simulink model "Sim6_lim_current_LCL"  (R2018b)
settings: Solver=ode1  StartTime=0.0  StopTime=5  FixedStep=Time_Step  MaxStep=1e-4  RelTol=1e-3
undefined symbols (not defined in the file): Bxx_GenericVoltageSource, C_line, Lg, Rg, Source_Lib, Theta0, Time_Step, Un, V0, VSC01_id0
libraries: powerlib x34, Control_Lib x7, powerlib_meascontrol x4, simulink x4
(part 1 of 2)
settings Model: Creator=Frederic_Colas  LastModifiedBy=fcolas
settings OptimizationCC: LifeSpan=inf
settings DebuggingCC: UnconnectedInputMsg=none  UnconnectedOutputMsg=none  UnconnectedLineMsg=none  SFExecutionAtInitializationDiag=none
settings HardwareCC: ProdBitPerSizeT=32  ProdBitPerPtrDiffT=32  ProdWordSize=32  ProdHWDeviceType=Specified
settings SFSimCC: SimUseLocalCustomCode=off
settings RTWCC: RTWUseLocalCustomCode=off
settings CodeAppCC: StateflowObjectComments=on
settings SimscapeCC: SimscapeNormalizeSystem=off

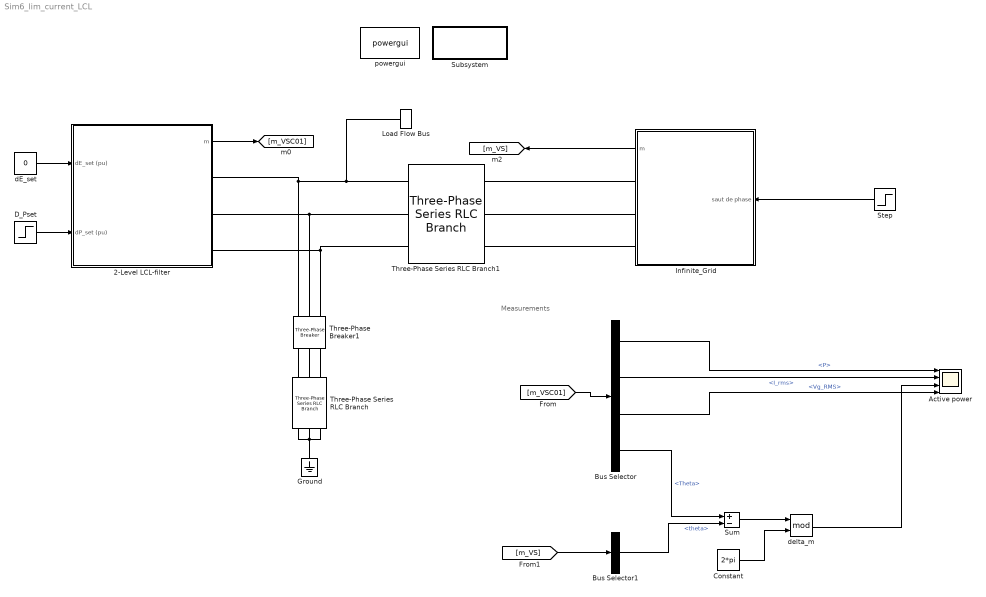
== system Sim6_lim_current_LCL ==
  note: Measurements
  2-Level LCL-filter : Subsystem  AncestorBlock=GFo_Lib/2-Level LCL-filter  mask(VSC){fn=50, Sn=1000e6, Pn=1000e6, Udcn=640e3, Time_Step=Time_Step, bridge_type=Average (no switches), fpwm=4e3, Un1=320e3, Un2=400e3, Rt_pu=0.005, Lt_pu=0.15, Rm_pu=500, Lm_pu=500, Lf_pu=0.15, Rf_pu=0.005, Cf_pu=0.066, H_DC=40, Tr_PLL=10, Val_Freq_Support=on, Val_gamma=on, R_percent=4, Rv=0.009, W_TVR=60, I_max_VI_pu=1.1, DX_DR=5, Kp_Rvi_pu=0.676, RLCL_D=0.7, f_damping=100, I_max_pu=1.15, Tr_I_max=10, Advanced=on, gainpopup=With Inertia, f_Inertia_Less=3, zeta_Inertia_Less=1, Param_Inertia=PI, H_GFo=5, zeta_GFo=0.7, LFpopup=PQ, P0=0.5, Q0=-1.3878e-17, V0=1.0022, Theta0=1.429}
      mask prompts: fn "Nominal Frequency (Hz)"; Sn "Nominal Apparent Power (VA)"; Pn "Nominal Power (W)"; Udcn "Nominal DC Voltage (V)"; Time_Step "Sample Time (s)"; bridge_type "Bridge Type"; fpwm "PWM frequency (Hz)"; Un1 "VSC side Nominal Ph-Ph Voltage (V)"; Un2 "Grid side Nominal Ph-Ph Voltage (V)"; Rt_pu "R (pu)"; Lt_pu "L (pu)"; Rm_pu "Rm (pu)"; Lm_pu "Lm (pu)"; Lf_pu "Lf (pu)"; Rf_pu "Rf (pu)"; Cf_pu "Cf (pu)"; H_DC "DC inertia (ms)"; Tr_PLL "Time response (ms)"; Val_Freq_Support "Frequency Support"; Val_gamma "gamma activation"; R_percent "Droop Gain (%)"; Rv "Damping Resistance (Rv)"; W_TVR "Dr filter"; I_max_VI_pu "Current Threshold (pu)"; Kp_Rvi_pu "Kp_Rvi"; RLCL_D "LC Damping Resistance (pu)"; f_damping "Cut-off Frequency (Hz)"; I_max_pu "I max (pu)"; Tr_I_max "Current Loop time response (ms)"; gainpopup "Strategy"; f_Inertia_Less "Bandwidth (Hz)"; zeta_Inertia_Less "Damping"; H_GFo "Inertia H (s)"; zeta_GFo "Damping Ratio"; P0 "Initial Active Power (pu)"; Q0 "Initial Reactive Power (pu)"; V0 "Initial Voltage (pu)"; Theta0 "Initial Angle (°)"
      mask init:
      | % Base values
      |     % 1 = VSC side
      |     % 2 = grid side
      |     fb = fn;
      |     Pb = Pn;
      |     cos_phi_n = Pn/Sn;
      |     Sb = Pb/cos_phi_n;
      |     Vn1 = Un1/sqrt(3);
      |     Vb1 = Vn1;
      |     Vn2 = Un2/sqrt(3);
      |     Vb2 = Vn2;
      |     Ib1 = Sb / (3*Vb1);
      |     Ib2 = Sb / (3*Vb2);
      |     Zb = (3*Vb1^2)/Sb;
      |     wb = 2*pi*fb;  wb_pu=1;
      |     Lb = Zb/wb;
      |     Cb = 1/(Zb*wb);
      |     
      | % Grid-Forming control tuning
      |     % Inertia Less
      |     wn_Inertia_Less = 2*pi*f_Inertia_Less;
      |     Ki_Inertia_Less = Lt_pu*wn_Inertia_Less^2/wb;
      |     Kp_Inertia_Less = 2*zeta_Inertia_Less*wn_Inertia_Less*Lt_pu/wb;
      |     
      |     % With Inertia
      |     Kc = 1/Lf_pu;
      |     Kg = 1/Lt_pu;
      |     %H_Gfo = 3;
      |     %wn = sqrt(wb*Kc*Kg/(2*H_Gfo*(Kc+Kg)));
      |     kp_GFo = zeta_GFo*sqrt(2*(Kc+Kg)/(H_GFo*wb*Kc*Kg));
      |     kd = 2*H_GFo*kp_GFo*Kc*wb;
      |   
      | % PLL derivation of the parameters
      |     wn_PLL=5/Tr_PLL;
      |     zeta_PLL = 1;
      |     Kp_PLL_pu = 2*zeta_PLL*wn_PLL/wb;
      |     Ki_PLL_pu = wn_PLL^2/wb;
      |     
      |     
      |     % VI calculation
      | 
      | 
      |   A_VI = (1 + 1/DX_DR^2);
      |   B_VI = 2*Lt_pu;
      |   C_VI = Lt_pu^2 - 1/I_max_VI_pu^2;
      |   
      |   Delta_VI = B_VI^2 - 4*A_VI*C_VI;
      |   
      |   X1_VI = (-B_VI + sqrt(Delta_VI))/(2*A_VI);
      |   Kp_Rvi_pu = X1_VI/(DX_DR*(-1+I_max_VI_pu));
      |   
      |   
      | % Set the chosen strategy
      |     if (gainpopup == 1)
      |         Chosen_Strategy = 1;
      |     elseif (gainpopup == 2)
      |         if (Param_Inertia == 1)
      |             Chosen_Strategy = 2;
      |         elseif (Param_Inertia == 2)
      |             Chosen_Strategy = 3;
      |         end
      |     end
      |     %Chosen_Strategy = 2;
      |     
      | % Set the frequency droop gain
      |     R = R_percent/100;
      | 
      | % Compute the delay compensation between control and power parts
      |     if (Time_Step == -1)
      |         Solver_Time_Step = 0;
      |     else
      |         Solver_Time_Step = Time_Step;
      |     end
      | 
      | % Compute Initial Voltage of VSC 
      | %   from steady-state output transformer model and Loadflow result
      |     
      |     %Initialize correctly the LoadFlow bus parameters connected to PCC
      |     VLF = V0;
      |     ThetaLF = Theta0;
      |     if (LFpopup == 'PQ')
      |         VLF = 1;
      |         ThetaLF = 0;
      |     elseif (LFpopup == 'PV')
      |         VLF = V0;
      |         ThetaLF = 0;        
      |     end
      |     %set_param([gcb '/Load Flow Bus'],'Vref',num2str(VLF),'Vangle',num2str(ThetaLF));
      | 
      |     % steady-state model of output transformer
      |     R1_pu = Rt_pu/2;
      |     L1_pu = Lt_pu/2;
      |     R2_pu = Rt_pu/2;
      |     L2_pu = Lt_pu/2;
      |     X1_pu = L1_pu;
      |     X2_pu = L2_pu;
      |     Xm_pu = Lm_pu;
      |     wb_pu = 1;
      |     
      |     Zm_pu = 1/(1/Rm_pu+1/(1i*Xm_pu));
      |     S0=P0+1i*Q0;
      |     I2 = conj(S0)/(V0);
      |     Vm = (R2_pu+1i*X2_pu)*I2 + V0;
      |     Im = Vm/Zm_pu;
      |     I1 = I2 + Im;
      |     V1 = (R1_pu+1i*X1_pu) * I1 + Vm;
      |     
      |     Eg0 = abs(V1); % compute initial Eg value
      |     Theta_m0 = angle(V1) * 180/pi+Theta0;
      |     
      |     %Steady-state model of LC Filter
      |     Is = I1 + 1i*Cf_pu*V1;
      |     Theta_Is = angle(Is) * 180/pi+Theta0;
      |     Vm = (1i*Lf_pu+Rf_pu)*Is+ V1;  %  
      |     
      | % Generate string to display LF results on Mask
      |     %str_tmp = fprintf("Vvsc0 = %d, Theta_vsc0 = %d°",Vvsc0,Theta_vsc0);
      |     mo = get_param(gcb,'MaskObject');
      |     mo.getDialogControl('LF_pcc_str').Prompt = ['V0 = ', num2str(V0),' pu, Angle = ', num2str(Theta0),'°'];
      |     mo.getDialogControl('LF_pcc_Power_str').Prompt = ['P0 = ', num2str(P0),' pu, Q0 = ', num2str(Q0),' pu'];
      |     %set_param([gcb],'LF_str',str_tmp);
      |  %GRD00_Theta0 = Theta0;
      |  % Initial current and voltage states calculation 
      |  
      | % Given Setpoint in PV bus
      |  
      | Vg0_d=V0*cos(Theta0*pi/180-Theta_m0*pi/180);
      | Vg0_q=V0*sin(Theta0*pi/180-Theta_m0*pi/180);
      | Vg0_dq = [Vg0_d ;Vg0_q; 0];
      |  
      | % Initial state of AC grid current : Ig0dq
      | 
      | Theta_I2 = angle(I2) * 180/pi + Theta0;
      | Ig0_d = abs(I2)*cos(Theta_I2*pi/180-Theta_m0*pi/180);
      | Ig0_q = abs(I2)*sin(Theta_I2*pi/180-Theta_m0*pi/180);
      | Ig0_dq = [Ig0_d; Ig0_q; 0];
      |  
      | % Initial state of capacitor voltage : eg0dq
      | 
      | Eg0_d = Eg0;
      | Eg0_q = 0;
      | Eg0_dq = [Eg0; 0; 0];
      |  
      | % Initial state of VSC Current : Is0dq
      | 
      | Is0_d = abs(Is) * cos(Theta_Is*pi/180-Theta_m0*pi/180);
      | Is0_q = abs(Is) * sin(Theta_Is*pi/180-Theta_m0*pi/180);
      | Is0_dq = [Is0_d; Is0_q; 0];
      | 
      | % Initial state of Modulation Voltage : Vm0dq
      | 
      | Vvsc0 = abs(Vm);
      | Theta_vsc0 = angle(Vm)*180/pi + Theta0;
      | Vm0_d = Vvsc0 * cos(Theta_vsc0*pi/180-Theta_m0*pi/180);
      | Vm0_q = Vvsc0 * sin(Theta_vsc0*pi/180-Theta_m0*pi/180);
      |  
      | Va0 = sqrt(2)*Vb1*Vvsc0*sin(Theta_vsc0*pi/180);
      | Vb0 = sqrt(2)*Vb1*Vvsc0*sin(Theta_vsc0*pi/180-2*pi/3);
      | Vc0 = sqrt(2)*Vb1*Vvsc0*sin(Theta_vsc0*pi/180+2*pi/3);
      | Vabc0 = [Va0 Vb0 Vc0];
      |  
      | mo.getDialogControl('LF_vsc_str').Prompt = ['V0 = ', num2str(Eg0),' pu, Angle = ', num2str(Theta_m0),'°'];
      settings: OpenFcn=|
      | NameStr = get_param(gcb,'Name');
      | open_system(gcbh, 'Mask');
      | 
      | h2AllOpenDlgs = DAStudio.ToolRoot.getOpenDialogs;
      | 
      | for i=1:length(h2AllOpenDlgs)
      |     try
      |          %disp(h2AllOpenDlgs(i).getSource.getBlock.Name);
      |         Dialog_block_name = h2AllOpenDlgs(i).getSource.getBlock.Name;
      |          %strcmp(Dialog_block_name, NameStr),
      |         if (strcmp(h2AllOpenDlgs(i).getSource.getBlock.Name, NameStr))
      |             iPos = h2AllOpenDlgs(i).position;
      |             h2AllOpenDlgs(i).position = [iPos(1)   iPos(2)   iPos(3)*1.6   iPos(4)];
      |         end
      |     end
      | end
      mask TypeOptions bridge_type: Average (no switches) | Detailed (switches included)
      mask Callback bridge_type:
      | % Get the mask parameter values. This is a cell
      | %   array of character vectors.
      | maskStr = get_param(gcb,'bridge_type');
      | p=Simulink.Mask.get(gcb);
      | 
      | % The pop-up menu is the first mask parameter.
      | %   Check the value selected in the pop-up
      | if strcmp(maskStr,'Average (no switches)'),
      | 
      |     % Set the visibility of both parameters on when
      |     %   User-defined is selected in the pop-up.
      |     p.getDialogControl('pwm_box').Visible='off';
      |     set_param([gcb '/Bridge_Model/Average'],'Commented','off');
      |     set_param([gcb '/Bridge_Model/Detailed'],'Commented','on');
      | 
      | 
      | elseif strcmp(maskStr,'Detailed (switches included)'),
      | 
      |     % Set the visibility of both parameters on when
      |     %   User-defined is selected in the pop-up.
      |     p.getDialogControl('pwm_box').Visible='on';
      |     set_param([gcb '/Bridge_Model/Average'],'Commented','on');
      |     set_param([gcb '/Bridge_Model/Detailed'],'Commented','off');
      | 
      | end
      mask Callback Advanced:
      | % Get the mask parameter values. This is a cell
      | %   array of character vectors.
      | maskStr = get_param(gcb,'Advanced');
      | p=Simulink.Mask.get(gcb);
      | 
      | % The pop-up menu is the first mask parameter.
      | %   Check the value selected in the pop-up
      | if strcmp(maskStr,'on'),
      | 
      |     % Set the visibility of both parameters on when
      |     %   User-defined is selected in the pop-up.
      |     p.getDialogControl('TVR').Visible='on';
      |     p.getDialogControl('TVI').Visible='on';
      |     p.getDialogControl('LC_Filter').Visible='on';
      |     p.getDialogControl('Current_Sat').Visible='on';
      |     %p.getDialogControl('Param_Strat_3').Visible='off';
      | 
      | 
      | else
      | 
      |     % Set the visibility of both parameters on when
      |     %   User-defined is selected in the pop-up.
      |     p.getDialogControl('TVR').Visible='off';
      |     p.getDialogControl('TVI').Visible='off';
      |     p.getDialogControl('LC_Filter').Visible='off';
      |     p.getDialogControl('Current_Sat').Visible='off';
      |     %p.getDialogControl('Param_Strat_3').Visible='off';
      | 
      | end
      mask TypeOptions gainpopup: Inertia Less | With Inertia
      mask Callback gainpopup:
      | % Get the mask parameter values. This is a cell
      | %   array of character vectors.
      | maskStr = get_param(gcb,'gainpopup');
      | p=Simulink.Mask.get(gcb);
      | 
      | % The pop-up menu is the first mask parameter.
      | %   Check the value selected in the pop-up
      | if strcmp(maskStr,'Inertia Less'),
      | 
      |     % Set the visibility of both parameters on when
      |     %   User-defined is selected in the pop-up.
      |     p.getDialogControl('No_Inertia').Visible='on';
      |     p.getDialogControl('Inertia').Visible='off';
      |     %p.getDialogControl('Param_Strat_3').Visible='off';
      | 
      | 
      | elseif strcmp(maskStr,'With Inertia'),
      | 
      |     % Set the visibility of both parameters on when
      |     %   User-defined is selected in the pop-up.
      |     p.getDialogControl('No_Inertia').Visible='off';
      |     p.getDialogControl('Inertia').Visible='on';
      |     %p.getDialogControl('Param_Strat_3').Visible='off';
      | 
      | 
      |     % Turn off the visibility of the Value field
      |     %   when User-defined is not selected.
      | 
      | else
      | 
      |     % Set the visibility of both parameters on when
      |     %   User-defined is selected in the pop-up.
      |     p.getDialogControl('No_Inertia').Visible='off';
      |     p.getDialogControl('Inertia').Visible='off';
      |     %p.getDialogControl('Param_Strat_3').Visible='off';
      | 
      | end
      mask TypeOptions Param_Inertia: VSM | PI
      mask TypeOptions LFpopup: Swing | PQ | PV
      mask Callback LFpopup:
      | % Get the mask parameter values. This is a cell
      | %   array of character vectors.
      | maskStr = get_param(gcb,'LFpopup');
      | p=Simulink.Mask.get(gcb);
      | 
      | % The pop-up menu is the first mask parameter.
      | %   Check the value selected in the pop-up
      | if strcmp(maskStr,'Swing'),
      | 
      |     % Set the visibility of both parameters on when
      |     %   User-defined is selected in the pop-up.
      |     p.getParameter('P0').Visible='off';
      |     p.getParameter('Q0').Visible='off';
      |     p.getParameter('V0').Visible='on';
      |     p.getParameter('Theta0').Visible='on';
      |     set_param([gcb '/Source_For_LF'],'BusType','swing');
      | 
      | elseif strcmp(maskStr,'PQ'),
      | 
      |     % Set the visibility of both parameters on when
      |     %   User-defined is selected in the pop-up.
      |     p.getParameter('P0').Visible='on';
      |     p.getParameter('Q0').Visible='on';
      |     %p.getParameter('V0').Value='1';
      |     %set_param(gcb,'V0','1');
      |     p.getParameter('V0').Visible='off';
      |     p.getParameter('Theta0').Visible='off';
      |     set_param([gcb '/Source_For_LF'],'BusType','PQ');
      | 
      |     % Turn off the visibility of the Value field
      |     %   when User-defined is not selected.
      | else
      | 
      |     % Set the visibility of both parameters on when
      |     %   User-defined is selected in the pop-up.
      |     p.getParameter('P0').Visible='on';
      |     p.getParameter('Q0').Visible='off';
      |     p.getParameter('V0').Visible='on';
      |     p.getParameter('Theta0').Visible='off';
      |     set_param([gcb '/Source_For_LF'],'BusType','PV');
      | 
      | end
      mask DialogControl Nominal_Param Prompt: Nominal Value
      mask DialogControl Container20 Prompt: Passive Components
      mask DialogControl Container31 Prompt: Transformer
      mask DialogControl Container32 Prompt: Filter
      mask DialogControl Container35 Prompt: DC Link
      mask DialogControl Control_Param Prompt: Control Parameter
      mask DialogControl Container13 Prompt: PLL
      mask DialogControl Container14 Prompt: Frequency Support
      mask DialogControl TVR Prompt: Transient Virtual Resistor
      mask DialogControl TVI Prompt: Virtual Impedance
      mask DialogControl LC_Filter Prompt: LC Filter
      mask DialogControl Current_Sat Prompt: Current Limitation
      mask DialogControl Container18 Prompt: Control Strategy
      mask DialogControl LF_Param Prompt: Loadflow
      mask DialogControl Control4 Prompt: Initial Operating Point
      mask DialogControl Container24 Prompt: VSC side
      mask DialogControl LF_vsc_str Prompt: V0 = 1.0076 pu, Angle = 5.6968°
      mask DialogControl Container25 Prompt: PCC
      mask DialogControl LF_pcc_str Prompt: V0 = 1.0022 pu, Angle = 1.429°
      mask DialogControl LF_pcc_Power_str Prompt: P0 = 0.5 pu, Q0 = -1.3878e-17 pu
      mask DialogControl UpdateLoadflow Prompt: Update Loadflow
      mask DialogControl UpdateLoadflow Callback: LoadFlow_VSC
      mask Display:
      | disp('LCL-Filter');
      | port_label('input',1,'dE_set (pu)');
      | port_label('input',2,'dP_set (pu)');
      | port_label('output',1,'m');
      | port_label('rconn',1,'A');
      | port_label('rconn',2,'B');
      | port_label('rconn',3,'C');
  Active power : Scope  NumInputPorts=4
  Bus Selector : BusSelector  OutputSignals=P,VI.I_rms,V.Vg_RMS,Theta
  Bus Selector1 : BusSelector  OutputSignals=Theta.theta
  Constant : Constant  Value=2*pi
  D_Pset : Step  After=0  SampleTime=0
  Ground : powerlib/Elements/Ground  LConnTagsString=a
  Infinite_Grid : Subsystem  AncestorBlock=Source_Lib/Bxx_GenericVoltageSource  mask(GenericVoltageSource){SourceNature_str=INFINITE, fn=50, Sn=1e9, Un=Un, LFpopup=Swing, P0=-498595539.7375, Q0=12437610.3184, V0_pu=1, U0=20000, Theta0_deg=0, H_s=5, DroopOnOff=on, R_percent=4, TN=1, TD=2}
      mask prompts: SourceNature_str "Nature of the voltage source"; fn "Nominal frequency fn [Hz]"; Sn "Nominal apparent power Sn [VA]"; Un "Nominal voltage Un [V RMS Ph2Ph]"; P0 "Active power P0 [W]"; Q0 "Reactive power Q0 [VAR]"; V0_pu "Initial pu voltage V0_pu [pu]"; U0 "Initial voltage U0 [Vrms Ph2Ph]"; Theta0_deg "Initial angle (°)"; H_s "Inertia H [s]"; DroopOnOff "Frequency DROOP activation"; R_percent "Droop gain Kp [%]"; TN "Network time constant Lead [s]"; TD "Network time constant Lag [s]"
      mask init:
      | % Update Name of LF bus for internal purpose
      | NameStr = [get_param(gcb,'Name')];% '_LF'];
      | set_param([gcb '/Load Flow Bus'],'ID',NameStr);  
      | 
      | % Base specification
      | fb = fn;                % [Hz] base frequency
      | Sb = Sn;                % [VA] base power
      | Ub = Un;                % [V] base ph2ph voltage
      | Vb = Un/sqrt(3);        % [V] base ph2N voltage
      | Ib = Sb/(3*Vb);         % [A] base current
      | Zb = Vb*Ib;             % [Ohm] base impedance
      | 
      | % Set the frequency droop gain
      | R = R_percent / 100;
      | 
      | %Initialize correctly the LoadFlow bus parameters connected to PCC
      |     VLF = V0_pu;
      |     ThetaLF = Theta0_deg;
      |     if (LFpopup == 'PQ')
      |         VLF = 1;
      |         ThetaLF = 0;
      |     elseif (LFpopup == 'PV')
      |         VLF = V0_pu;
      |         ThetaLF = 0;        
      |     end
      |     set_param([gcb '/Load Flow Bus'],'Vref',num2str(VLF),'Vangle',num2str(ThetaLF));
      | 
      | 
      | % Update mask display:
      | % mo = get_param(gcb,'MaskObject');
      mask TypeOptions SourceNature_str: INFINITE | INERTIAL
      mask Callback SourceNature_str:
      | % Get the mask parameter values. This is a cell
      | %   array of character vectors.
      | maskStr = get_param(gcb,'SourceNature_str');
      | p=Simulink.Mask.get(gcb);
      | 
      | % The pop-up menu is the first mask parameter.
      | %   Check the value selected in the pop-up
      | if strcmp(maskStr,'INFINITE')
      |    p.getParameter('H_s').Visible='off';
      |    p.getParameter('DroopOnOff').Visible='off';
      |    DroopOnOff = 'off';
      |    p.getParameter('R_percent').Visible='off';
      |    p.getParameter('TN').Visible='off';
      |    p.getParameter('TD').Visible='off';
      |    set_param([gcb '/SourceNature'],'Value','1')
      | else
      |    p.getParameter('H_s').Visible='on';
      |    p.getParameter('DroopOnOff').Visible='on';
      |    DroopOnOff = 'on';
      |    p.getParameter('R_percent').Visible='on';
      |    p.getParameter('TN').Visible='on';
      |    p.getParameter('TD').Visible='on';
      |    set_param([gcb '/SourceNature'],'Value','2')
      | end
      mask TypeOptions LFpopup: Swing | PQ | PV
      mask Callback LFpopup:
      | % Get the mask parameter values. This is a cell
      | %   array of character vectors.
      | maskStr = get_param(gcb,'LFpopup');
      | p=Simulink.Mask.get(gcb);
      | 
      | % The pop-up menu is the first mask parameter.
      | %   Check the value selected in the pop-up
      | if strcmp(maskStr,'Swing'),
      | 
      |     % Set the visibility of both parameters on when
      |     %   User-defined is selected in the pop-up.
      |     p.getParameter('P0').Enabled='off';
      |     p.getParameter('Q0').Enabled='off';
      |     p.getParameter('V0_pu').Enabled='on';
      |     p.getParameter('U0').Enabled='off';
      |     p.getParameter('Theta0_deg').Enabled='off';
      |     set_param([gcb '/Source_For_LF'],'BusType','swing');
      | 
      | elseif strcmp(maskStr,'PQ'),
      | 
      |     % Set the visibility of both parameters on when
      |     %   User-defined is selected in the pop-up.
      |     p.getParameter('P0').Enabled='on';
      |     p.getParameter('Q0').Enabled='on';
      |     p.getParameter('V0_pu').Enabled='off';
      |     p.getParameter('U0').Enabled='off';
      |     p.getParameter('Theta0_deg').Enabled='off';
      |     set_param([gcb '/Source_For_LF'],'BusType','PQ');
      | 
      |     % Turn off the visibility of the Value field
      |     %   when User-defined is not selected.
      | else
      | 
      |     % Set the visibility of both parameters on when
      |     %   User-defined is selected in the pop-up.
      |     p.getParameter('P0').Enabled='on';
      |     p.getParameter('Q0').Enabled='off';
      |     p.getParameter('V0_pu').Enabled='on';
      |     p.getParameter('U0').Enabled='off';
      |     p.getParameter('Theta0_deg').Enabled='off';
      |     set_param([gcb '/Source_For_LF'],'BusType','PV');
      | 
      | end
      mask Callback DroopOnOff:
      | % Get the mask parameter values. This is a cell
      | %   array of character vectors.
      | maskStr = get_param(gcb,'DroopOnOff');
      | p=Simulink.Mask.get(gcb);
      | 
      | if strcmp(maskStr,'on'),
      |     p.getParameter('R_percent').Enabled='on';
      | else
      |     p.getParameter('R_percent').Enabled='off';
      | end
      mask DialogControl Container2 Prompt: Nominal specification (for base definition)
      mask DialogControl Container3 Prompt: Loadflow specification
      mask DialogControl InertialConfig Prompt: Inertial source configuration
  Load Flow Bus : powerlib/Measurements/Load Flow Bus  LConnTagsString=a  Phases=single  Connectors=on one side  ID=BUS_1  Vbase=Un  Vref=1  Vangle=0  VLF=1.002  VLFb=1  VLFc=1  angleLF=1.429  angleLFb=0  angleLFc=0
  Step : Step  After=0  SampleTime=0
  Subsystem : Subsystem
      settings: OpenFcn=LoadFlow_VSC
      mask Display: color('blue'),disp('Update Loadflow')
  Sum : Sum  Inputs=+-
  Three-Phase Series RLC Branch : powerlib/Elements/Three-Phase Series RLC Branch  LConnTagsString=A|B|C  RConnTagsString=A|B|C  BranchType=R  Resistance=0.1  Inductance=1e-3  Capacitance=1e-6  Measurements=None
  Three-Phase Series RLC Branch1 : powerlib/Elements/Three-Phase Series RLC Branch  LConnTagsString=A|B|C  RConnTagsString=A|B|C  BranchType=RL  Resistance=Rg  Inductance=Lg  Capacitance=1e-6  Measurements=None
  Three-Phase Breaker1 : powerlib/Elements/Three-Phase Breaker  InitialState=open  SwitchA=on  SwitchB=on  SwitchC=on  SwitchTimes=[0.2 0.8]  External=off  BreakerResistance=0.01  SnubberResistance=1e6  SnubberCapacitance=inf  Measurements=None
  dE_set : Constant  Value=0
  delta_m : Math  Operator=mod  SaturateOnIntegerOverflow=on
  powergui : powerlib/powergui  Priority=1  SimulationMode=Discrete  SampleTime=Time_Step  frequency=60  Iterations=50  frequencyindice=50  Pbase=1000000000  ErrMax=1e-6  UnitsV=kV  UnitsW=MW  buscounter=0  FunctionMessages=off  echomessages=off  EnableUseOfTLC=off  CurrentSourceSwitches=off  DisableSnubberDevices=off  DisableRonSwitches=off  DisableVfSwitches=off  DisplayEquations=off  AutomaticDiscreteSolvers=off  SolverType=Tustin/Backward Euler (TBE)  Interpol=off  ExternalGateDelay=off  methode=off  Ts=100  x0status=blocks  SPID=on  SwTol=0  HookPort=off  NonlinearTolerance=1e-4  nMaxIteration=100  ContinueOnMaxIteration=off  RestoreLinks=warning  ResistiveCurrentMeasurement=off  Frange=[0:2:500]  Ylog=off  Xlog=on  ShowGrid=off  save=off  variable=ZData  structure=0  ZoomFFT=off  StartTime=0.0  cycles=1  DisplayStyle=1  fundamental=60  FreqAxis=off  MaxFrequency=1000  frequencyindicesteady=1  RmsSteady=1  display=off
  wires:
  dE_set/1 -> 2-Level LCL-filter/1(dE_set (pu))
  D_Pset/1 -> 2-Level LCL-filter/2(dP_set (pu))
  2-Level LCL-filter/1(m) -> [m_VSC01]
  Infinite_Grid/1(m) -> [m_VS]
  Bus Selector/1 -> Active power/1  "<P>"
  Bus Selector1/1 -> Sum/2  "<theta>"
  Bus Selector/2 -> Active power/2  "<I_rms>"
  [m_VSC01] -> Bus Selector/1
  [m_VS] -> Bus Selector1/1
  Bus Selector/4 -> Sum/1  "<Theta>"
  Step/1 -> Infinite_Grid/1(saut de phase)
  Sum/1 -> delta_m/1
  delta_m/1 -> Active power/3
  Constant/1 -> delta_m/2
  Bus Selector/3 -> Active power/4  "<Vg_RMS>"
  connections:
  Three-Phase Breaker1/RConn1 -- 2-Level LCL-filter/RConn1 -- Load Flow Bus/LConn1 -- Three-Phase Series RLC Branch1/LConn1
  Three-Phase Breaker1/RConn3 -- 2-Level LCL-filter/RConn3 -- Three-Phase Series RLC Branch1/LConn3
  Three-Phase Breaker1/RConn2 -- 2-Level LCL-filter/RConn2 -- Three-Phase Series RLC Branch1/LConn2
  Infinite_Grid/RConn1 -- Three-Phase Series RLC Branch1/RConn1
  Infinite_Grid/RConn2 -- Three-Phase Series RLC Branch1/RConn2
  Infinite_Grid/RConn3 -- Three-Phase Series RLC Branch1/RConn3
  Three-Phase Series RLC Branch/RConn1 -- Three-Phase Series RLC Branch/RConn2 -- Three-Phase Series RLC Branch/RConn3 -- Ground/LConn1
  Three-Phase Series RLC Branch/LConn3 -- Three-Phase Breaker1/LConn3
  Three-Phase Breaker1/LConn2 -- Three-Phase Series RLC Branch/LConn2
  Three-Phase Series RLC Branch/LConn1 -- Three-Phase Breaker1/LConn1

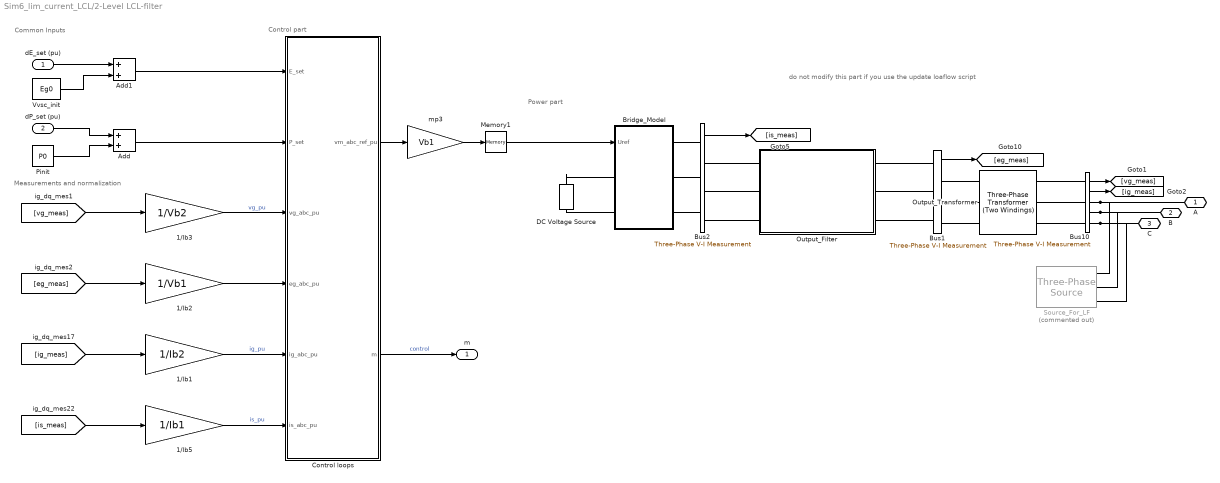
== system Sim6_lim_current_LCL/2-Level LCL-filter ==
  note: Common Inputs
  note: Power part
  note: Measurements and normalization
  note: Control part
  note: do not modify this part if you use the update loaflow script
  dE_set (pu) : Inport
  dP_set (pu) : Inport  Port=2
  1/Ib1 : Gain  Gain=1/Ib2
  1/Ib2 : Gain  Gain=1/Vb1
  1/Ib3 : Gain  Gain=1/Vb2
  1/Ib5 : Gain  Gain=1/Ib1
  Add : Sum
  Add1 : Sum
  Bridge_Model : Subsystem
  Bus1 : powerlib/Measurements/Three-Phase V-I Measurement  VoltageMeasurement=phase-to-ground  SetLabelV=off  LabelV=Vabc  Vpu=off  VpuLL=off  CurrentMeasurement=no  SetLabelI=off  LabelI=Iabc  Ipu=off  Pbase=100e6  Vbase=500e3  OutputType=Complex  PhasorSimulation=off  PSBequivalent=0
  Bus10 : powerlib/Measurements/Three-Phase V-I Measurement  VoltageMeasurement=phase-to-ground  SetLabelV=off  LabelV=Vabc  Vpu=off  VpuLL=off  CurrentMeasurement=yes  SetLabelI=off  LabelI=Iabc  Ipu=off  Pbase=100e6  Vbase=500e3  OutputType=Complex  PhasorSimulation=off  PSBequivalent=0
  Bus2 : powerlib/Measurements/Three-Phase V-I Measurement  VoltageMeasurement=no  SetLabelV=off  LabelV=Vabc  Vpu=off  VpuLL=off  CurrentMeasurement=yes  SetLabelI=off  LabelI=Iabc  Ipu=off  Pbase=100e6  Vbase=500e3  OutputType=Complex  PhasorSimulation=off  PSBequivalent=0
  Control loops : Subsystem
  DC Voltage Source : powerlib/Electrical Sources/DC Voltage Source  Amplitude=Udcn  Measurements=Voltage
  Memory1 : Memory  InitialCondition=[Va0 Vb0 Vc0]
  Output_Filter : Subsystem
  Output_Transformer : powerlib/Elements/Three-Phase Transformer (Two Windings)  Winding1Connection=Yg  Winding2Connection=Yg  CoreType=Three single-phase transformers  SetSaturation=off  Hysteresis=off  DataFile='hysteresis'  SetInitialFlux=off  Measurements=None  UNITS=pu  NominalPower=[Sn , fb]  Winding1=[Un1 , Rt_pu/2 , Lt_pu/2]  Winding2=[Un2 , Rt_pu/2 , Lt_pu/2]  Rm=Rm_pu  Lm=Lm_pu  L0=0.5  Saturation=[ 0,0 ; 0.0024,1.2 ; 1.0,1.52 ]  InitialFluxes=[-1.0109960716468 0.506091473811006 0.504904597835851]  BreakLoop=off  DiscreteSolver=Trapezoidal iterative  DataType=off  TransfoNumber=1
  Pinit : Constant  Value=P0
  Source_For_LF : powerlib/Electrical Sources/Three-Phase Source  Commented=on  InternalConnection=Yg  VoltagePhases=off  Voltage=(400000)*1.00218  PhaseAngle=1.429  Voltage_phases=[25e3 25e3 25e3]/sqrt(3)  PhaseAngles_phases=[0 -120 +120]  Frequency=fb  NonIdealSource=off  SpecifyImpedance=off  Resistance=0  Inductance=0  ShortCircuitLevel=100e6  BaseVoltage=Un  XRratio=7  BusType=PQ  Pref=P0*Sb  Qref=Q0*Sb  Prefabc=[10e3, 10e3, 10e3]  Qrefabc=[0, 0, 0]  Qmin=-inf  Qmax=inf
  Vvsc_init : Constant  Value=Eg0
  mp3 : Gain  Gain=Vb1
  A : PMIOPort  Side=Right
  B : PMIOPort  Port=2  Side=Right
  C : PMIOPort  Port=3  Side=Right
  m : Outport  VectorParamsAs1DForOutWhenUnconnected=off
  wires:
  [is_meas] -> 1/Ib5/1
  [ig_meas] -> 1/Ib1/1
  [eg_meas] -> 1/Ib2/1
  [vg_meas] -> 1/Ib3/1
  Memory1/1 -> Bridge_Model/1(Uref)
  Control loops/1(vm_abc_ref_pu) -> mp3/1
  1/Ib5/1 -> Control loops/6(is_abc_pu)  "is_pu"
  1/Ib2/1 -> Control loops/4(eg_abc_pu)
  Control loops/2(m) -> m/1  "control"
  1/Ib3/1 -> Control loops/3(vg_abc_pu)  "vg_pu"
  1/Ib1/1 -> Control loops/5(ig_abc_pu)  "ig_pu"
  Bus10/2 -> [ig_meas]
  mp3/1 -> Memory1/1
  Bus2/1 -> [is_meas]
  Bus10/1 -> [vg_meas]
  dP_set (pu)/1 -> Add/1
  Pinit/1 -> Add/2
  Vvsc_init/1 -> Add1/2
  Add1/1 -> Control loops/1(E_set)
  Bus1/1 -> [eg_meas]
  dE_set (pu)/1 -> Add1/1
  Add/1 -> Control loops/2(P_set)
  connections:
  Bus2/RConn3 -- Output_Filter/LConn3
  Bus2/RConn2 -- Output_Filter/LConn2
  Bus2/RConn1 -- Output_Filter/LConn1
  Bus2/LConn3 -- Bridge_Model/RConn3
  Bus2/LConn2 -- Bridge_Model/RConn2
  Bus2/LConn1 -- Bridge_Model/RConn1
  Bus10/RConn1 -- Source_For_LF/RConn1 -- A/RConn1
  Bus10/RConn2 -- Source_For_LF/RConn2 -- B/RConn1
  Bus10/RConn3 -- Source_For_LF/RConn3 -- C/RConn1
  Bus10/LConn3 -- Output_Transformer/RConn3
  Bus10/LConn2 -- Output_Transformer/RConn2
  Bus10/LConn1 -- Output_Transformer/RConn1
  Bus1/RConn3 -- Output_Transformer/LConn3
  Bus1/RConn2 -- Output_Transformer/LConn2
  Output_Transformer/LConn1 -- Bus1/RConn1
  Bus1/LConn3 -- Output_Filter/RConn3
  Bus1/LConn2 -- Output_Filter/RConn2
  Bus1/LConn1 -- Output_Filter/RConn1
  Bridge_Model/LConn2 -- DC Voltage Source/LConn1
  DC Voltage Source/RConn1 -- Bridge_Model/LConn1

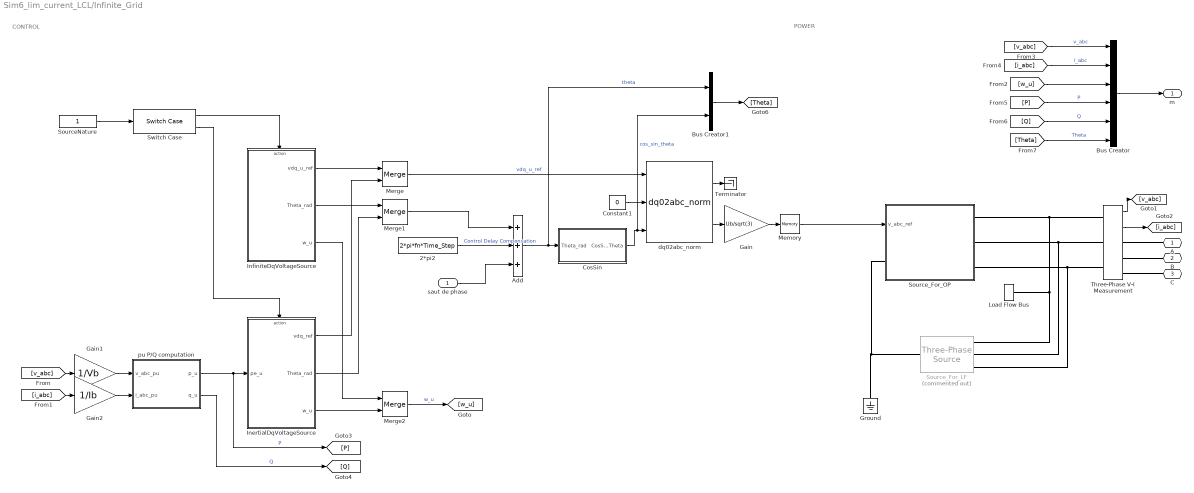
== system Sim6_lim_current_LCL/Infinite_Grid ==
  note: POWER
  note: CONTROL
  saut de phase : Inport
  " pu P/Q computation" : Subsystem  DialogController=POWERSYS.PowerSysDialog
  2*pi2 : Constant  Value=2*pi*fn*Time_Step
  Add : Sum  Inputs=+++
  Bus Creator : BusCreator  Inputs=6
  Bus Creator1 : BusCreator  Inputs=2
  Constant1 : Constant  Value=0
  CosSin : Subsystem
  Gain : Gain  Gain=Ub/sqrt(3)
  Gain1 : Gain  Gain=1/Vb
  Gain2 : Gain  Gain=1/Ib
  Ground : powerlib/Elements/Ground  LConnTagsString=a
  InertialDqVoltageSource : Subsystem  TreatAsAtomicUnit=on
  InfiniteDqVoltageSource : Subsystem  TreatAsAtomicUnit=on
  Load Flow Bus : powerlib/Measurements/Load Flow Bus  LConnTagsString=a  Phases=single  Connectors=on one side  ID=Infinite_Grid  Vbase=Un  Vref=1  Vangle=0  VLF=1  VLFb=1  VLFc=1  angleLF=0  angleLFb=0  angleLFc=0
  Memory : Memory
  Merge : Merge
  Merge1 : Merge
  Merge2 : Merge
  SourceNature : Constant
  Source_For_LF : powerlib/Electrical Sources/Three-Phase Source  Commented=on  InternalConnection=Yn  VoltagePhases=off  Voltage=(400000)*1  PhaseAngle=0  Voltage_phases=[25e3 25e3 25e3]/sqrt(3)  PhaseAngles_phases=[0 -120 +120]  Frequency=fb  NonIdealSource=off  SpecifyImpedance=off  Resistance=0  Inductance=0  ShortCircuitLevel=100e6  BaseVoltage=Un  XRratio=7  BusType=swing  Pref=P0  Qref=Q0  Prefabc=[10e3, 10e3, 10e3]  Qrefabc=[0, 0, 0]  Qmin=-inf  Qmax=inf
  Source_For_OP : Subsystem
  Switch Case : SwitchCase  CaseConditions={1, 2}  ShowDefaultCase=off
  Terminator : Terminator
  Three-Phase V-I Measurement : powerlib/Measurements/Three-Phase V-I Measurement  VoltageMeasurement=phase-to-ground  SetLabelV=off  LabelV=v_abc  Vpu=off  VpuLL=off  CurrentMeasurement=yes  SetLabelI=off  LabelI=i_abc  Ipu=off  Pbase=100e6  Vbase=500e3  OutputType=Complex  PhasorSimulation=off  PSBequivalent=0
  dq02abc_norm : Control_Lib/dq02abc_norm  referenceAxisMode=Reference axis at 90 degrees behind phase_a  baseUpdateGain=sqrt(3)
      settings: SourceProductName=VSC_Lib
  A : PMIOPort  Side=Right
  B : PMIOPort  Port=2  Side=Right
  C : PMIOPort  Port=3  Side=Right
  m : Outport  VectorParamsAs1DForOutWhenUnconnected=off
  wires:
  [Q] -> Bus Creator/5  "Q"
  [P] -> Bus Creator/4  "P"
  Three-Phase V-I Measurement/2 -> [i_abc]
  Three-Phase V-I Measurement/1 -> [v_abc]
  Bus Creator/1 -> m/1
  Merge2/1 -> [w_u]  "w_u"
  InfiniteDqVoltageSource/3(w_u) -> Merge2/1
  [w_u] -> Bus Creator/3
  [i_abc] -> Bus Creator/2  "i_abc"
  [v_abc] -> Bus Creator/1  "v_abc"
  InertialDqVoltageSource/3(w_u) -> Merge2/2
  2*pi2/1 -> Add/2  "Control Delay Compensation"
  Merge1/1 -> Add/1
  Add/1 -> Bus Creator1/1, CosSin/1(Theta_rad)  "theta"
  Memory/1 -> Source_For_OP/1(v_abc_ref)
  " pu P/Q computation"/1(p_u) -> InertialDqVoltageSource/1(pe_u), [P]  "P"
  " pu P/Q computation"/2(q_u) -> [Q]  "Q"
  CosSin/1(CosSinTheta) -> Bus Creator1/2, dq02abc_norm/3  "cos_sin_theta"
  Gain2/1 -> " pu P/Q computation"/2(i_abc_pu)
  Gain1/1 -> " pu P/Q computation"/1(v_abc_pu)
  [i_abc] -> Gain2/1
  [v_abc] -> Gain1/1
  Switch Case/2 -> InertialDqVoltageSource/Action
  InertialDqVoltageSource/2(Theta_rad) -> Merge1/2
  InfiniteDqVoltageSource/2(Theta_rad) -> Merge1/1
  Merge/1 -> dq02abc_norm/1  "vdq_u_ref"
  InertialDqVoltageSource/1(vdq_ref) -> Merge/2
  InfiniteDqVoltageSource/1(vdq_u_ref) -> Merge/1
  Switch Case/1 -> InfiniteDqVoltageSource/Action
  SourceNature/1 -> Switch Case/1
  Gain/1 -> Memory/1
  dq02abc_norm/1 -> Terminator/1
  Constant1/1 -> dq02abc_norm/2
  dq02abc_norm/2 -> Gain/1
  Bus Creator1/1 -> [Theta]
  [Theta] -> Bus Creator/6  "Theta"
  saut de phase/1 -> Add/3
  connections:
  Three-Phase V-I Measurement/RConn3 -- C/RConn1
  Three-Phase V-I Measurement/RConn2 -- B/RConn1
  Three-Phase V-I Measurement/RConn1 -- A/RConn1
  Three-Phase V-I Measurement/LConn1 -- Load Flow Bus/LConn1 -- Source_For_LF/RConn1 -- Source_For_OP/RConn1
  Source_For_OP/RConn3 -- Three-Phase V-I Measurement/LConn3 -- Source_For_LF/RConn3
  Source_For_LF/LConn1 -- Ground/LConn1 -- Source_For_OP/LConn1
  Source_For_OP/RConn2 -- Three-Phase V-I Measurement/LConn2 -- Source_For_LF/RConn2

== system Sim6_lim_current_LCL/Subsystem ==

== system Sim6_lim_current_LCL/2-Level LCL-filter/Bridge_Model ==
  Uref : Inport
  Average : powerlib/Power Electronics/Universal Bridge  Arms=3  SnubberResistance=1e5  SnubberCapacitance=inf  Device=Average-model based VSC  Ron=1e-3  Lon=0  ForwardVoltages="[  0  0  ]"  ForwardVoltage=0  GTOparameters=[ 10e-6 , 20e-6 ]  IGBTparameters=[ 1e-6 , 2e-6 ]  Measurements=None  Measurements_2=None  converterType=Rectifier
  Constant : Constant
  Detailed : Subsystem  Commented=on
  Memory : Memory
  NOT1 : Logic  Operator=NOT  IconShape=distinctive  AllPortsSameDT=off  OutDataTypeStr=boolean
  Saturation : Saturate  UpperLimit=1  LowerLimit=-1
  Three-Phase Breaker1 : powerlib/Elements/Three-Phase Breaker  InitialState=closed  SwitchA=on  SwitchB=on  SwitchC=on  SwitchTimes="[4/60  10/60]"  External=on  BreakerResistance=0.001  SnubberResistance=1e6  SnubberCapacitance=inf  Measurements=None
  Three-Phase Breaker2 : powerlib/Elements/Three-Phase Breaker  InitialState=open  SwitchA=on  SwitchB=on  SwitchC=on  SwitchTimes="[4/60  10/60]"  External=on  BreakerResistance=0.001  SnubberResistance=1e6  SnubberCapacitance=inf  Measurements=None
  Three-Phase Source : powerlib/Electrical Sources/Three-Phase Source  InternalConnection=Yg  VoltagePhases=off  Voltage=Vvsc0*Un1  PhaseAngle=Theta_vsc0  Voltage_phases=[25e3 25e3 25e3]/sqrt(3)  PhaseAngles_phases=[0 -120 +120]  Frequency=fb  NonIdealSource=off  SpecifyImpedance=off  Resistance=0  Inductance=0  ShortCircuitLevel=100e6  BaseVoltage=VSC01_Un1  XRratio=7  BusType=swing  Pref=0.3  Qref=0  Prefabc=[10e3, 10e3, 10e3]  Qrefabc=[0, 0, 0]  Qmin=-Inf  Qmax=Inf
  mp3 : Gain  Gain=2/Udcn
  PhA : PMIOPort  Side=Right
  PhB : PMIOPort  Port=2  Side=Right
  PhC : PMIOPort  Port=3  Side=Right
  Vdc+ : PMIOPort  Port=4  Side=Left
  Vdc- : PMIOPort  Port=5  Side=Left
  wires:
  Saturation/1 -> Detailed/1(Urref), Average/1
  mp3/1 -> Saturation/1
  Constant/1 -> Memory/1
  Memory/1 -> NOT1/1, Three-Phase Breaker2/1
  NOT1/1 -> Three-Phase Breaker1/1
  Uref/1 -> mp3/1
  connections:
  Three-Phase Breaker2/LConn1 -- Three-Phase Breaker1/LConn1 -- PhA/RConn1
  Three-Phase Breaker2/LConn2 -- Three-Phase Breaker1/LConn2 -- PhB/RConn1
  Three-Phase Breaker2/LConn3 -- Three-Phase Breaker1/LConn3 -- PhC/RConn1
  Three-Phase Breaker2/RConn1 -- Average/LConn1 -- Detailed/LConn1
  Three-Phase Breaker2/RConn2 -- Detailed/LConn2 -- Average/LConn2
  Three-Phase Source/RConn1 -- Three-Phase Breaker1/RConn1
  Three-Phase Source/RConn2 -- Three-Phase Breaker1/RConn2
  Three-Phase Source/RConn3 -- Three-Phase Breaker1/RConn3
  Average/RConn1 -- Detailed/RConn1 -- Vdc+/RConn1
  Detailed/RConn2 -- Average/RConn2 -- Vdc-/RConn1
  Three-Phase Breaker2/RConn3 -- Detailed/LConn3 -- Average/LConn3

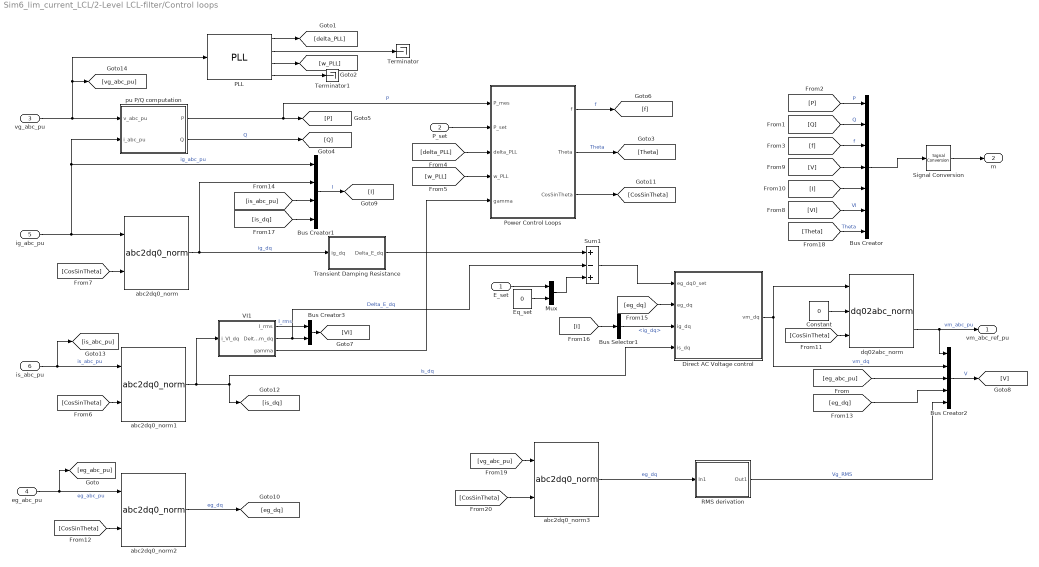
== system Sim6_lim_current_LCL/2-Level LCL-filter/Control loops ==
  E_set : Inport
  P_set : Inport  Port=2
  vg_abc_pu : Inport  Port=3
  eg_abc_pu : Inport  Port=4
  ig_abc_pu : Inport  Port=5
  is_abc_pu : Inport  Port=6
  " pu P/Q computation" : Subsystem  DialogController=POWERSYS.PowerSysDialog
  Bus Creator : BusCreator  Inputs=7
  Bus Creator1 : BusCreator  Inputs=4
  Bus Creator2 : BusCreator  Inputs=5
  Bus Creator3 : BusCreator  Inputs=2
  Bus Selector1 : BusSelector  OutputSignals=ig_dq
  Constant : Constant  Value=0
  Direct AC Voltage control : Subsystem
  Eq_set : Constant  Value=0
  Mux : Mux  Inputs=2
  PLL : Control_Lib/PLL  fb=fb  Tr_PLL=Tr_PLL  Theta0=Theta0
      settings: SourceProductName=VSC4SPS
  Power Control Loops : Subsystem
  RMS derivation : Subsystem
  Signal Conversion : SignalConversion  OverrideOpt=off
  Sum1 : Sum  Inputs=+-+
  Terminator : Terminator
  Terminator1 : Terminator
  Transient Damping Resistance : Subsystem
  VI1 : Subsystem
  abc2dq0_norm{,1..3} (4 alike) : Control_Lib/abc2dq0_norm  referenceAxisMode=Reference axis at 90 degrees behind phase_a  baseUpdateGain=1/sqrt(3)
      settings: SourceProductName=VSC4SPS
  dq02abc_norm : Control_Lib/dq02abc_norm  referenceAxisMode=Reference axis at 90 degrees behind phase_a  baseUpdateGain=sqrt(3)
      settings: SourceProductName=VSC4SPS
  vm_abc_ref_pu : Outport  PortDimensions=3  VectorParamsAs1DForOutWhenUnconnected=off
  m : Outport  Port=2  VectorParamsAs1DForOutWhenUnconnected=off
  wires:
  PLL/4 -> Terminator1/1
  PLL/2 -> Terminator/1
  Constant/1 -> dq02abc_norm/2
  Power Control Loops/3(CosSinTheta) -> [CosSinTheta]
  PLL/3 -> [w_PLL]
  PLL/1 -> [delta_PLL]
  Sum1/1 -> Direct AC Voltage control/1(eg_dq0_set)
  [I] -> Bus Selector1/1
  Bus Selector1/1 -> Direct AC Voltage control/3(ig_dq)  "<ig_dq>"
  Bus Creator2/1 -> [V]  "V"
  [CosSinTheta] -> dq02abc_norm/3
  dq02abc_norm/2 -> vm_abc_ref_pu/1, Bus Creator2/1  "vm_abc_pu"
  Direct AC Voltage control/1(vm_dq) -> Bus Creator2/2, dq02abc_norm/1  "vm_dq"
  [eg_dq] -> Direct AC Voltage control/2(eg_dq)
  eg_abc_pu/1 -> [eg_abc_pu], abc2dq0_norm2/1  "eg_abc_pu"
  is_abc_pu/1 -> abc2dq0_norm1/1, [is_abc_pu]  "is_abc_pu"
  abc2dq0_norm2/2 -> [eg_dq]  "eg_dq"
  [CosSinTheta] -> abc2dq0_norm2/2
  abc2dq0_norm1/2 -> VI1/1(i_VI_dq), [is_dq], Direct AC Voltage control/4(is_dq)  "is_dq"
  vg_abc_pu/1 -> [vg_abc_pu], PLL/1, " pu P/Q computation"/1(v_abc_pu)
  [CosSinTheta] -> abc2dq0_norm1/2
  [I] -> Bus Creator/5
  Bus Creator1/1 -> [I]  "I"
  Bus Creator/1 -> Signal Conversion/1
  [VI] -> Bus Creator/6  "VI"
  [V] -> Bus Creator/4
  Eq_set/1 -> Mux/2
  VI1/1(I_rms) -> Bus Creator3/1  "I_rms"
  Transient Damping Resistance/1("Delta_E_dq ") -> Sum1/1
  VI1/2(Delta_vm_dq) -> Sum1/2, Bus Creator3/2  "Delta_E_dq"
  [CosSinTheta] -> abc2dq0_norm/2
  Power Control Loops/2(Theta) -> [Theta]  "Theta"
  abc2dq0_norm/2 -> Transient Damping Resistance/1(ig_dq), Bus Creator1/2  "ig_dq"
  ig_abc_pu/1 -> " pu P/Q computation"/2(i_abc_pu), Bus Creator1/1, abc2dq0_norm/1  "ig_abc_pu"
  " pu P/Q computation"/1(P) -> [P], Power Control Loops/1(P_mes)  "P"
  Power Control Loops/1(f) -> [f]  "f"
  [w_PLL] -> Power Control Loops/4(w_PLL)
  P_set/1 -> Power Control Loops/2(P_set)
  [delta_PLL] -> Power Control Loops/3(delta_PLL)
  " pu P/Q computation"/2(Q) -> [Q]  "Q"
  E_set/1 -> Mux/1
  [f] -> Bus Creator/3  "f"
  [Q] -> Bus Creator/2  "Q"
  [P] -> Bus Creator/1  "P"
  Signal Conversion/1 -> m/1
  Bus Creator3/1 -> [VI]
  [eg_abc_pu] -> Bus Creator2/3
  [eg_dq] -> Bus Creator2/4
  [is_abc_pu] -> Bus Creator1/3
  [is_dq] -> Bus Creator1/4
  [Theta] -> Bus Creator/7  "Theta"
  VI1/3(gamma) -> Power Control Loops/5(gamma)
  Mux/1 -> Sum1/3
  RMS derivation/1(Out1) -> Bus Creator2/5  "Vg_RMS"
  [vg_abc_pu] -> abc2dq0_norm3/1
  [CosSinTheta] -> abc2dq0_norm3/2
  abc2dq0_norm3/2 -> RMS derivation/1(In1)  "eg_dq"

== system Sim6_lim_current_LCL/2-Level LCL-filter/Output_Filter ==
  Filter capacitance : powerlib/Elements/Three-Phase Series RLC Branch  LConnTagsString=A|B|C  RConnTagsString=A|B|C  BranchType=C  Resistance=0  Inductance=C_line(1)  Capacitance=Cf_pu*Cb  Measurements=None
  Filter inductance : powerlib/Elements/Three-Phase Series RLC Branch  LConnTagsString=A|B|C  RConnTagsString=A|B|C  BranchType=RL  Resistance=Rf_pu*Zb  Inductance=Lf_pu*Lb  Capacitance=1e-6  Measurements=None
  Ground : powerlib/Elements/Ground  LConnTagsString=a
  A : PMIOPort  Side=Left
  a : PMIOPort  Port=2  Side=Right
  B : PMIOPort  Port=3  Side=Left
  b : PMIOPort  Port=4  Side=Right
  C : PMIOPort  Port=5  Side=Left
  c : PMIOPort  Port=6  Side=Right
  connections:
  Ground/LConn1 -- Filter capacitance/RConn1 -- Filter capacitance/RConn3 -- Filter capacitance/RConn2
  b/RConn1 -- Filter capacitance/LConn2 -- Filter inductance/RConn2
  Filter inductance/LConn1 -- A/RConn1
  Filter inductance/LConn3 -- C/RConn1
  Filter inductance/LConn2 -- B/RConn1
  c/RConn1 -- Filter capacitance/LConn3 -- Filter inductance/RConn3
  a/RConn1 -- Filter capacitance/LConn1 -- Filter inductance/RConn1

== system Sim6_lim_current_LCL/Infinite_Grid/ pu P//Q computation ==
  v_abc_pu : Inport  PortDimensions=3
  i_abc_pu : Inport  Port=2  PortDimensions=3
  Demux : Demux  Outputs=3
      settings: DisplayOption=none
  Mux : Mux  Inputs=3
  Product1 : Product  InputSameDT=on  SaturateOnIntegerOverflow=on  OutDataTypeStr=Inherit: Same as first input
  Product3 : Product  InputSameDT=on  SaturateOnIntegerOverflow=on  OutDataTypeStr=Inherit: Same as first input
  Sum : Sum  Inputs=+-  InputSameDT=on  SaturateOnIntegerOverflow=on  OutDataTypeStr=Inherit: Same as first input
  Sum1 : Sum  Inputs=1  InputSameDT=on  SaturateOnIntegerOverflow=on  OutDataTypeStr=Inherit: Same as first input
  Sum4 : Sum  Inputs=1  InputSameDT=on  SaturateOnIntegerOverflow=on  OutDataTypeStr=Inherit: Same as first input
  Sum5 : Sum  Inputs=+-  InputSameDT=on  SaturateOnIntegerOverflow=on  OutDataTypeStr=Inherit: Same as first input
  Sum6 : Sum  Inputs=+-  InputSameDT=on  SaturateOnIntegerOverflow=on  OutDataTypeStr=Inherit: Same as first input
  pu->V : Gain  Gain=1/sqrt(3)  SaturateOnIntegerOverflow=on  OutDataTypeStr=Inherit: Same as input  ParamDataTypeStr=Inherit: Same as input
  pu->V1 : Gain  Gain=1/3  SaturateOnIntegerOverflow=on  OutDataTypeStr=Inherit: Same as input  ParamDataTypeStr=Inherit: Same as input
  pu->V2 : Gain  Gain=1/3  SaturateOnIntegerOverflow=on  OutDataTypeStr=Inherit: Same as input  ParamDataTypeStr=Inherit: Same as input
  p_u : Outport  VectorParamsAs1DForOutWhenUnconnected=off
  q_u : Outport  Port=2  VectorParamsAs1DForOutWhenUnconnected=off
  wires:
  pu->V/1 -> pu->V2/1  "Q"
  Mux/1 -> Product3/1
  Sum6/1 -> Mux/2
  Sum5/1 -> Mux/1
  Sum/1 -> Mux/3
  Demux/3 -> Sum6/1, Sum5/2
  Demux/2 -> Sum5/1, Sum/2
  Demux/1 -> Sum6/2, Sum/1
  Sum4/1 -> pu->V1/1
  i_abc_pu/1 -> Product3/2, Product1/2
  v_abc_pu/1 -> Demux/1, Product1/1
  Product1/1 -> Sum4/1
  Product3/1 -> Sum1/1
  Sum1/1 -> pu->V/1
  pu->V1/1 -> p_u/1
  pu->V2/1 -> q_u/1

== system Sim6_lim_current_LCL/Infinite_Grid/CosSin ==
  Theta_rad : Inport
  Mux : Mux  Inputs=2
  Trigonometric Function : Trigonometry
  Trigonometric Function1 : Trigonometry  Operator=cos
  CosSinTheta : Outport  VectorParamsAs1DForOutWhenUnconnected=off
  wires:
  Trigonometric Function1/1 -> Mux/1
  Mux/1 -> CosSinTheta/1
  Trigonometric Function/1 -> Mux/2
  Theta_rad/1 -> Trigonometric Function1/1, Trigonometric Function/1

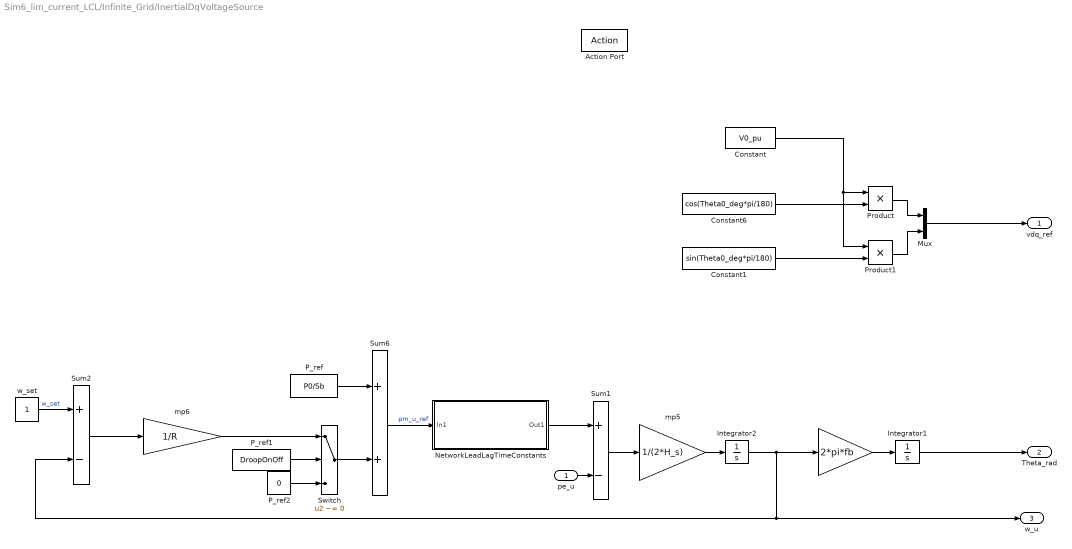
== system Sim6_lim_current_LCL/Infinite_Grid/InertialDqVoltageSource ==
  pe_u : Inport
  Action Port : ActionPort
  " " : Gain  Gain=2*pi*fb
  Constant : Constant  Value=V0_pu
  Constant1 : Constant  Value=sin(Theta0_deg*pi/180)
  Constant6 : Constant  Value=cos(Theta0_deg*pi/180)
  Integrator1 : Integrator
  Integrator2 : Integrator  InitialCondition=1
  Mux : Mux  Inputs=2
  NetworkLeadLagTimeConstants : Subsystem
  P_ref : Constant  Value=P0/Sb
  P_ref1 : Constant  Value=DroopOnOff
  P_ref2 : Constant  Value=0
  Product : Product
  Product1 : Product
  Sum1 : Sum  Inputs=+-
  Sum2 : Sum  Inputs=+-
  Sum6 : Sum
  Switch : Switch  Criteria=u2 ~= 0
  mp5 : Gain  Gain=1/(2*H_s)
  mp6 : Gain  Gain=1/R
  w_set : Constant
  vdq_ref : Outport  VectorParamsAs1DForOutWhenUnconnected=off
  Theta_rad : Outport  Port=2  VectorParamsAs1DForOutWhenUnconnected=off
  w_u : Outport  Port=3  VectorParamsAs1DForOutWhenUnconnected=off
  wires:
  P_ref2/1 -> Switch/3
  mp6/1 -> Switch/1
  Switch/1 -> Sum6/2
  P_ref1/1 -> Switch/2
  NetworkLeadLagTimeConstants/1(Out1) -> Sum1/1
  Mux/1 -> vdq_ref/1
  Product/1 -> Mux/1
  Product1/1 -> Mux/2
  Constant/1 -> Product/1, Product1/1
  Constant6/1 -> Product/2
  Constant1/1 -> Product1/2
  Integrator1/1 -> Theta_rad/1
  w_set/1 -> Sum2/1  "w_set"
  pe_u/1 -> Sum1/2
  " "/1 -> Integrator1/1
  Sum1/1 -> mp5/1
  Sum2/1 -> mp6/1
  P_ref/1 -> Sum6/1
  Integrator2/1 -> " "/1, Sum2/2, w_u/1
  Sum6/1 -> NetworkLeadLagTimeConstants/1(In1)  "pm_u_ref"
  mp5/1 -> Integrator2/1

== system Sim6_lim_current_LCL/Infinite_Grid/InfiniteDqVoltageSource ==
  Action Port : ActionPort
  Constant : Constant  Value=V0_pu
  Constant1 : Constant  Value=sin(Theta0_deg*pi/180)
  Constant4 : Constant
  Constant6 : Constant  Value=cos(Theta0_deg*pi/180)
  Gain : Gain  Gain=2*pi*fn
  Integrator : Integrator
  Mux : Mux  Inputs=2
  Product : Product
  Product1 : Product
  vdq_u_ref : Outport  VectorParamsAs1DForOutWhenUnconnected=off
  Theta_rad : Outport  Port=2  VectorParamsAs1DForOutWhenUnconnected=off
  w_u : Outport  Port=3  VectorParamsAs1DForOutWhenUnconnected=off
  wires:
  Constant4/1 -> Gain/1, w_u/1
  Mux/1 -> vdq_u_ref/1
  Integrator/1 -> Theta_rad/1
  Product1/1 -> Mux/2
  Constant/1 -> Product/1, Product1/1
  Constant6/1 -> Product/2
  Product/1 -> Mux/1
  Gain/1 -> Integrator/1
  Constant1/1 -> Product1/2

== system Sim6_lim_current_LCL/Infinite_Grid/Source_For_OP ==
  v_abc_ref : Inport
  Controlled Voltage Source1 : powerlib/Electrical Sources/Controlled Voltage Source  Initialize=off  Source_Type=AC  Amplitude=V0*Ub*sqrt(2/3)*sin(Theta0)  Phase=(Theta0*180/pi)  Frequency=fb  Measurements=None
  Controlled Voltage Source2 : powerlib/Electrical Sources/Controlled Voltage Source  Initialize=off  Source_Type=AC  Amplitude=V0*Ub*sqrt(2/3)*sin(Theta0-2*pi/3)  Phase=(Theta0*180/pi)-120  Frequency=fb  Measurements=None
  Controlled Voltage Source3 : powerlib/Electrical Sources/Controlled Voltage Source  Initialize=off  Source_Type=AC  Amplitude=V0*Ub*sqrt(2/3)*sin(Theta0-4*pi/3)  Phase=(Theta0*180/pi)+120  Frequency=fb  Measurements=None
  Demux : Demux  Outputs=3
  Step : Step  Time=1e-9  SampleTime=0
  Subsystem3 : Subsystem
  Three-Phase Source1 : powerlib/Electrical Sources/Three-Phase Source  InternalConnection=Yn  VoltagePhases=off  Voltage=V0_pu*Ub  PhaseAngle=Theta0_deg  Voltage_phases=[25e3 25e3 25e3]/sqrt(3)  PhaseAngles_phases=[0 -120 +120]  Frequency=fb  NonIdealSource=off  SpecifyImpedance=off  Resistance=0.8929  Inductance=16.58e-3  ShortCircuitLevel=100e6  BaseVoltage=25e3  XRratio=7  BusType=swing  Pref=10e3  Qref=0  Prefabc=[10e3, 10e3, 10e3]  Qrefabc=[0, 0, 0]  Qmin=-inf  Qmax=inf
  A : PMIOPort  Side=Right
  B : PMIOPort  Port=2  Side=Right
  C : PMIOPort  Port=3  Side=Right
  N : PMIOPort  Port=4  Side=Left
  wires:
  Step/1 -> Subsystem3/1(switch)
  Demux/3 -> Controlled Voltage Source3/1
  Demux/1 -> Controlled Voltage Source1/1
  v_abc_ref/1 -> Demux/1
  Demux/2 -> Controlled Voltage Source2/1
  connections:
  Three-Phase Source1/RConn3 -- Subsystem3/LConn6
  Three-Phase Source1/RConn2 -- Subsystem3/LConn5
  Three-Phase Source1/RConn1 -- Subsystem3/LConn4
  Controlled Voltage Source3/RConn1 -- Subsystem3/LConn3
  Controlled Voltage Source2/RConn1 -- Subsystem3/LConn2
  Controlled Voltage Source1/RConn1 -- Subsystem3/LConn1
  Subsystem3/RConn3 -- C/RConn1
  Subsystem3/RConn2 -- B/RConn1
  Subsystem3/RConn1 -- A/RConn1
  Controlled Voltage Source1/LConn1 -- Controlled Voltage Source2/LConn1 -- N/RConn1 -- Three-Phase Source1/LConn1 -- Controlled Voltage Source3/LConn1
